simulink model "Test_Byte_Multiplexer_8_to_1"  (R2023a)
settings: Solver=ode45  StartTime=0.0  StopTime=len  RelTol=1e-3  EnableMultiTasking=on
libraries: Miscellaneous x9, simulink x1, Byte_Multiplexers_Lib x1
settings Model: Creator=N  LastModifiedBy=Jozko Mrkvicka
settings SolverCC: AlgebraicLoopSolver=TrustRegion
settings DataIOCC: SaveFormat=Array  ReturnWorkspaceOutputs=off
settings OptimizationCC: LifeSpan=inf
settings DebuggingCC: UnconnectedInputMsg=warning  UnconnectedOutputMsg=warning  UnconnectedLineMsg=warning  SFUnexpectedBacktrackingDiag=warning  SFNoUnconditionalDefaultTransitionDiag=warning  ArithmeticOperatorsInVariantConditions=warning
settings HardwareCC: ProdWordSize=32
settings ModelReferenceCC: EnableRefExpFcnMdlSchedulingChecks=on
settings SFSimCC: SimUseLocalCustomCode=off  CustomCodeUndefinedFunction=UseInterfaceOnly
settings RTWCC: RTWUseLocalCustomCode=off
settings CodeAppCC: StateflowObjectComments=on
settings GRTTargetCC: TargetLangStandard=C89/C90 (ANSI)
settings ConfigComp: CovMetricSettings=dw  CovSaveCumulativeToWorkspaceVar=on  CovSaveSingleToWorkspaceVar=on  CovExternalEMLEnable=off

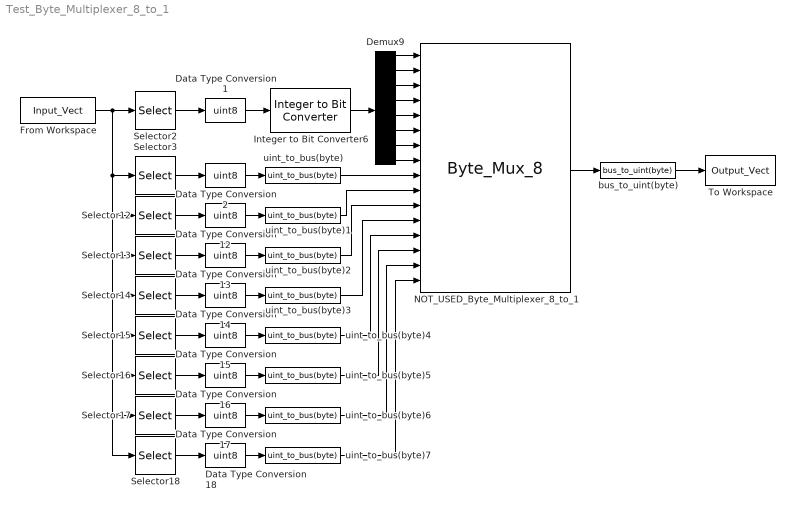
== system Test_Byte_Multiplexer_8_to_1 ==
  Data Type Conversion{1..2,12..18} (9 alike) : DataTypeConversion  OutDataTypeStr=uint8  SaturateOnIntegerOverflow=off  RndMeth=Floor
  Demux9 : Demux  Outputs=8
  From Workspace : FromWorkspace  VariableName=Input_Vect  SampleTime=1  Interpolate=off  ZeroCross=off  OutputAfterFinalValue=Holding final value
  Integer to Bit Converter6 : simulink/Logic and Bit Operations/Integer to Bit Converter  nbits=8  signedInputValues=Unsigned  bitOrder=MSB first  outDtype=boolean
      settings: LibrarySourceBlock=|
      | commutil2/Integer to Bit
      | Converter
  NOT_USED_Byte_Multiplexer_8_to_1 : Byte_Multiplexers_Lib/Byte_Mux_8  SystemSampleTime=-1  VariantActivationTime=update diagram  Latency=0  AutoFrameSizeCalculation=off
  Selector12 : Selector  IndexMode=Zero-based  InputPortWidth=9  IndexOptions=Index vector (dialog)  Indices=2  OutputSizes=1
  Selector13 : Selector  IndexMode=Zero-based  InputPortWidth=9  IndexOptions=Index vector (dialog)  Indices=3  OutputSizes=1
  Selector14 : Selector  IndexMode=Zero-based  InputPortWidth=9  IndexOptions=Index vector (dialog)  Indices=4  OutputSizes=1
  Selector15 : Selector  IndexMode=Zero-based  InputPortWidth=9  IndexOptions=Index vector (dialog)  Indices=5  OutputSizes=1
  Selector16 : Selector  IndexMode=Zero-based  InputPortWidth=9  IndexOptions=Index vector (dialog)  Indices=6  OutputSizes=1
  Selector17 : Selector  IndexMode=Zero-based  InputPortWidth=9  IndexOptions=Index vector (dialog)  Indices=7  OutputSizes=1
  Selector18 : Selector  IndexMode=Zero-based  InputPortWidth=9  IndexOptions=Index vector (dialog)  Indices=8  OutputSizes=1
  Selector2 : Selector  IndexMode=Zero-based  InputPortWidth=9  SampleTime=1  IndexOptions=Index vector (dialog)  Indices=0  OutputSizes=1
  Selector3 : Selector  IndexMode=Zero-based  InputPortWidth=9  IndexOptions=Index vector (dialog)  Indices=1  OutputSizes=1
  To Workspace : ToWorkspace  VariableName=Output_Vect  SampleTime=1
  bus_to_uint(byte) : Miscellaneous/bus_to_uint(byte)  SystemSampleTime=-1  VariantActivationTime=update diagram  Latency=0  AutoFrameSizeCalculation=off
  uint_to_bus(byte){,1..7} (8 alike) : Miscellaneous/uint_to_bus(byte)  SystemSampleTime=-1  VariantActivationTime=update diagram  Latency=0  AutoFrameSizeCalculation=off
  wires:
  NOT_USED_Byte_Multiplexer_8_to_1/1 -> bus_to_uint(byte)/1
  Demux9/1 -> NOT_USED_Byte_Multiplexer_8_to_1/1
  Demux9/2 -> NOT_USED_Byte_Multiplexer_8_to_1/2
  Demux9/3 -> NOT_USED_Byte_Multiplexer_8_to_1/3
  Integer to Bit Converter6/1 -> Demux9/1
  From Workspace/1 -> Selector12/1, Selector13/1, Selector14/1, Selector15/1, Selector16/1, Selector17/1, Selector18/1, Selector3/1, Selector2/1
  Selector2/1 -> Data Type Conversion1/1
  Selector3/1 -> Data Type Conversion2/1
  Data Type Conversion1/1 -> Integer to Bit Converter6/1
  Data Type Conversion2/1 -> uint_to_bus(byte)/1
  Selector12/1 -> Data Type Conversion12/1
  Selector13/1 -> Data Type Conversion13/1
  Selector14/1 -> Data Type Conversion14/1
  Selector15/1 -> Data Type Conversion15/1
  Selector16/1 -> Data Type Conversion16/1
  Selector17/1 -> Data Type Conversion17/1
  Selector18/1 -> Data Type Conversion18/1
  Data Type Conversion12/1 -> uint_to_bus(byte)1/1
  Data Type Conversion13/1 -> uint_to_bus(byte)2/1
  Data Type Conversion14/1 -> uint_to_bus(byte)3/1
  Data Type Conversion15/1 -> uint_to_bus(byte)4/1
  Data Type Conversion16/1 -> uint_to_bus(byte)5/1
  Data Type Conversion17/1 -> uint_to_bus(byte)6/1
  Data Type Conversion18/1 -> uint_to_bus(byte)7/1
  Demux9/8 -> NOT_USED_Byte_Multiplexer_8_to_1/8
  Demux9/4 -> NOT_USED_Byte_Multiplexer_8_to_1/4
  Demux9/5 -> NOT_USED_Byte_Multiplexer_8_to_1/5
  Demux9/6 -> NOT_USED_Byte_Multiplexer_8_to_1/6
  Demux9/7 -> NOT_USED_Byte_Multiplexer_8_to_1/7
  bus_to_uint(byte)/1 -> To Workspace/1
  uint_to_bus(byte)/1 -> NOT_USED_Byte_Multiplexer_8_to_1/9
  uint_to_bus(byte)1/1 -> NOT_USED_Byte_Multiplexer_8_to_1/10
  uint_to_bus(byte)2/1 -> NOT_USED_Byte_Multiplexer_8_to_1/11
  uint_to_bus(byte)3/1 -> NOT_USED_Byte_Multiplexer_8_to_1/12
  uint_to_bus(byte)4/1 -> NOT_USED_Byte_Multiplexer_8_to_1/13
  uint_to_bus(byte)5/1 -> NOT_USED_Byte_Multiplexer_8_to_1/14
  uint_to_bus(byte)6/1 -> NOT_USED_Byte_Multiplexer_8_to_1/15
  uint_to_bus(byte)7/1 -> NOT_USED_Byte_Multiplexer_8_to_1/16
